simulink library "avionics_lib"  (Simulink 6.6)
libraries: avionics_lib x1, avionics_T2_lib x1, avionics_S2_lib x1, simulink x1
settings Model: Creator=amurch  LastModifiedBy=amurch

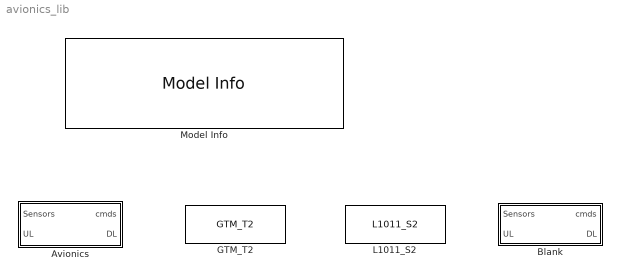
== system avionics_lib ==
  Avionics : Subsystem  BlockChoice=L1011_S2
      settings: TemplateBlock=self  MemberBlocks=Blank,GTM_T2,L1011_S2
  Blank : Subsystem
  GTM_T2 : avionics_T2_lib/GTM_T2  SystemSampleTime=-1
  L1011_S2 : avionics_S2_lib/L1011_S2  SystemSampleTime=-1
  Model Info : simulink/Model-Wide Utilities/Model Info  SystemSampleTime=-1  InitialBlockCM=None  BlockCM=None  Frame=on  DisplayStringWithTags=|  HorizontalTextAlignment=Center  LeftAlignmentValue=0.5  SourceBlockDiagram=avionics_lib  TagMaxNumber=20
      | Avionics Library
      | %<ModelVersion>
      | Las modified by %<LastModifiedBy> on %<LastModificationDate>

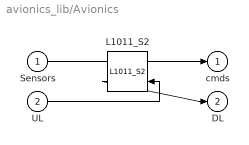
== system avionics_lib/Avionics ==
  Sensors : Inport
  UL : Inport  Port=2
  L1011_S2 : avionics_lib/L1011_S2  Orientation=left  SystemSampleTime=-1
  cmds : Outport
  DL : Outport  Port=2
  wires:
  Sensors/1 -> L1011_S2/1
  UL/1 -> L1011_S2/2
  L1011_S2/1 -> cmds/1
  L1011_S2/2 -> DL/1

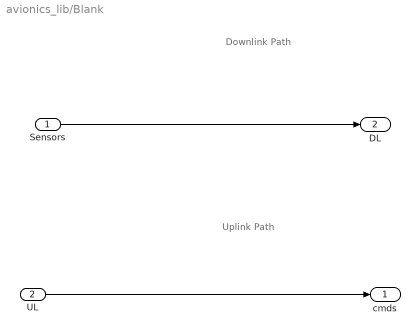
== system avionics_lib/Blank ==
  note: Uplink Path
  note: Downlink Path
  Sensors : Inport
  UL : Inport  Port=2
  cmds : Outport
  DL : Outport  Port=2
  wires:
  Sensors/1 -> DL/1
  UL/1 -> cmds/1
